simulink model "EMG_simulation_simulink"  (R2019a)
settings: Solver=VariableStepAuto  StartTime=0.0  StopTime=180  RelTol=1e-3
libraries: dsparch4 x1
settings Model: Creator=patri  LastModifiedBy=patri

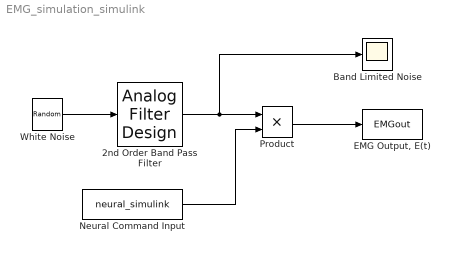
== system EMG_simulation_simulink ==
  2nd Order Band Pass Filter : dsparch4/Analog Filter Design  method=Butterworth  filttype=Bandpass  N=2  Wlo=62.83  Whi=3141.59  Rp=2  Rs=40
  Band Limited Noise : Scope
  "EMG Output, E(t)" : ToWorkspace  VariableName=EMGout  SampleTime=0.001
  Neural Command Input : FromWorkspace  VariableName=neural_simulink  SampleTime=0.001
  Product : Product
  White Noise : UniformRandomNumber  Minimum=-6.2e-4  Maximum=6.2e-4  SampleTime=0.001
  wires:
  Neural Command Input/1 -> Product/2
  2nd Order Band Pass Filter/1 -> Product/1, Band Limited Noise/1
  White Noise/1 -> 2nd Order Band Pass Filter/1
  Product/1 -> "EMG Output, E(t)"/1
